simulink library "ddm"  (R2021b)
settings: Solver=VariableStepAuto  StartTime=0.0  StopTime=10.0  RelTol=1e-3
undefined symbols (not defined in the file or in its folder): ENUM_ADASACCSTA_ERROR, ENUM_ADASACCSTA_OFF, ENUM_ADASACCSTA_STANDBY, ENUM_ADASISASTA_OFF, ENUM_ALLOWMOV_ALLOWREADY, ENUM_APS, ENUM_BRKSTA_ERROR, ENUM_BRKSTA_OFF, ENUM_BRKSTA_ON, ENUM_BRKSW_INVALID, ENUM_BRKSW_OFF, ENUM_BRKSW_ON, ENUM_CHGPREACTERRSTA_OBCPRE, ENUM_DCDCFAULTSTA_ANYFAULTLV1, ENUM_DCDCFAULTSTA_ANYFAULTLV2, ENUM_DRIVETRAIN_AWD, ENUM_DRIVETRAIN_FWD, ENUM_DRIVETRAIN_RWD, ENUM_DRSEATSTA_INVALID, ENUM_EDUDRTSTA_NORMAL, ENUM_EPBSTA_APPLIED, ENUM_EPBSTA_RELEASED, ENUM_HVBATTREADYPRE_READY, ENUM_MCUWARN_LV0, ENUM_MCUWARN_LV1, ENUM_MCUWARN_LV2, ENUM_MCUWARN_LV3, ENUM_MCUWARN_NOERROR, ENUM_OBCFAULTSTA_ANYFAULT, ENUM_PAS_R2F2, ENUM_PDFAULT_BATTPDFAIL, ENUM_PDFAULT_DCDCDISABLE, ENUM_PDFAULT_MCUDISABLE, ENUM_PDFAULT_MCUDISCHRG, ENUM_POWERSTA_OFF, ENUM_POWERSTA_ON, ENUM_POWERSTA_READY, ENUM_POWERSTA_STANDBY, ENUM_PRESSINDI_LOW, ENUM_PUFAULT_BATTUPFAIL, ENUM_PUFAULT_DCDCENABLEFAIL, ENUM_PUFAULT_PRECHRGCHKFAIL, ENUM_PUFAULT_SAFETYCHKFAIL, ENUM_PUSTATE_COMPLETED, ENUM_PWRSTASW_OFF, ENUM_PWRSTASW_OFFA, ENUM_PWRSTASW_OFFCHVCHRG, ENUM_PWRSTASW_OFFCLVCHRG, ENUM_PWRSTASW_ON, ENUM_PWRSTASW_ONHVCHRG, ENUM_PWRSTASW_READY, ENUM_PWRSTASW_STANDBY, ENUM_RANGESTA_12IN, ENUM_SHIFTCOMMAND_D, ENUM_SHIFTCOMMAND_N, ENUM_SHIFTCOMMAND_P, ENUM_SHIFTCOMMAND_R, ENUM_VEHMALFUNLV_2ND, ENUM_VEHMALFUNLV_3RD, ENUM_VEHMALFUNLV_4TH ... (+835)
libraries: hcu_lib x750, $bdroot x12, simulink x5
(part 11 of 28)

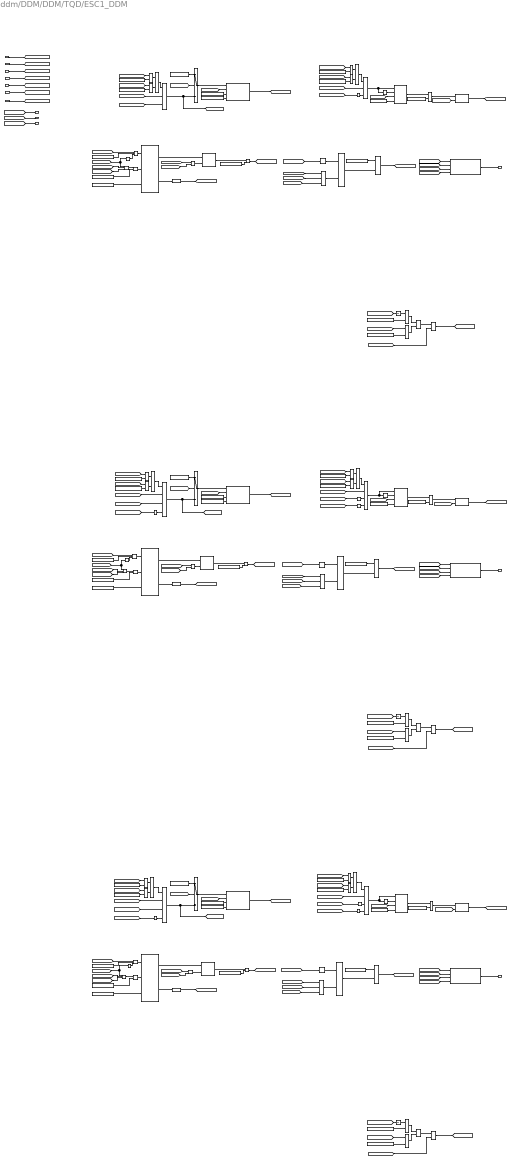
== system ddm/DDM/DDM/TQD/ESC1_DDM ==
  note: ESC1 Lost Comm (ESC1NoCom)
  note: ESC1 Rolling Count Error (ESC1RCErr)
  note: ESC1 CheckSum Error (ESC1CSErr)
  task_time_s : Inport
  VPMM_SysPwrSta_enum : Inport  Port=2
  No_CAN1_BUS_OFF : Inport  Port=3
  VDDM_ESC1NoCom_flg : Inport  Port=4
  VDDM_ESC1RCErr_flg : Inport  Port=5
  VDDM_ESC1CSErr_flg : Inport  Port=6
  DTC_clear_request : Inport  Port=7
  Constant{1,4,6,11,16..17} (6 alike) : Constant  Value=ENUM_PWRSTASW_READY
  Constant10 : Constant  Value=KDDM_ESC1RCErrDFSSW_flg
  Constant12 : Constant  Value=FALSE
  Constant13 : Constant  Value=KDDM_ESC1RCErrDTC_cnt
  Constant14 : Constant  Value=KDDM_ESC1RCErrPassTO_s
  Constant{2..3,5,7,15,19} (6 alike) : Constant  Value=ENUM_PWRSTASW_ON
  Constant18 : Constant  Value=KDDM_ESC1NoComDFSSW_flg
  Constant25 : Constant  Value=KDDM_ESC1RCErrDetTO_s
  Constant27 : Constant  Value=FALSE
  Constant28 : Constant  Value=KDDM_ESC1NoComDTC_cnt
  Constant29 : Constant  Value=KDDM_ESC1NoComPassTO_s
  Constant30 : Constant  Value=KDDM_ESC1NoComDetTO_s
  Constant31 : Constant  Value=ENUM_POWERSTA_OFF
  Constant32 : Constant  Value=ENUM_POWERSTA_STANDBY
  Constant33 : Constant  Value=KDDM_ESC1RCErrDetSW_flg
  Constant34 : Constant  Value=KDDM_ESC1RCErrPassSW_flg
  Constant35 : Constant  Value=KDDM_ESC1RCErrPassTO_s
  Constant36 : Constant  Value=KDDM_ESC1CSErrCFSSW_flg
  Constant37 : Constant  Value=KDDM_ESC1CSErrDTC_cnt
  Constant39 : Constant  Value=KDDM_ESC1CSErrDFSSW_flg
  Constant41 : Constant  Value=FALSE
  Constant42 : Constant  Value=KDDM_ESC1CSErrDTC_cnt
  Constant43 : Constant  Value=KDDM_ESC1CSErrPassTO_s
  Constant44 : Constant  Value=KDDM_ESC1CSErrDetTO_s
  Constant46 : Constant  Value=ENUM_POWERSTA_OFF
  Constant47 : Constant  Value=ENUM_POWERSTA_STANDBY
  Constant48 : Constant  Value=KDDM_ESC1CSErrDetSW_flg
  Constant49 : Constant  Value=ENUM_POWERSTA_OFF
  Constant50 : Constant  Value=KDDM_ESC1CSErrPassSW_flg
  Constant51 : Constant  Value=KDDM_ESC1CSErrPassTO_s
  Constant52 : Constant  Value=ENUM_POWERSTA_STANDBY
  Constant53 : Constant  Value=KDDM_ESC1NoComDetSW_flg
  Constant54 : Constant  Value=KDDM_ESC1NoComPassSW_flg
  Constant55 : Constant  Value=KDDM_ESC1NoComPassTO_s
  Constant56 : Constant  Value=KDDM_ESC1RCErrCFSSW_flg
  Constant57 : Constant  Value=KDDM_ESC1RCErrDTC_cnt
  Constant8 : Constant  Value=KDDM_ESC1NoComCFSSW_flg
  Constant9 : Constant  Value=KDDM_ESC1NoComDTC_cnt
  DTC_Couter2 : hcu_lib/Basic_Blocks/DTC_Couter
  DTC_Couter3 : hcu_lib/Basic_Blocks/DTC_Couter
  DTC_Couter4 : hcu_lib/Basic_Blocks/DTC_Couter
  DTC_Info1 : hcu_lib/Basic_Blocks/DTC_Info
  DTC_Info2 : hcu_lib/Basic_Blocks/DTC_Info
  DTC_Info3 : hcu_lib/Basic_Blocks/DTC_Info
  Data Type Conversion1 : DataTypeConversion  OutDataTypeStr=uint8
  Data Type Conversion3 : DataTypeConversion  OutDataTypeStr=uint8
  Data Type Conversion4 : DataTypeConversion  OutDataTypeStr=uint8
  Equal{1..14,16..18,22} (18 alike) : RelationalOperator  Operator===  OutDataTypeStr=boolean  RndMeth=Simplest
  Equal15 : RelationalOperator  OutDataTypeStr=boolean  RndMeth=Simplest
  Equal20 : RelationalOperator  OutDataTypeStr=boolean  RndMeth=Simplest
  Equal21 : RelationalOperator  OutDataTypeStr=boolean  RndMeth=Simplest
  Logical Operator{1..3,6..7,9..10,15,17,31,34,36} (12 alike) : Logic  Operator=OR  AllPortsSameDT=off  OutDataTypeStr=boolean
  Logical Operator{11..14,16,18..19,26,30,37,41,45,53} (13 alike) : Logic  Operator=NOT  AllPortsSameDT=off  OutDataTypeStr=boolean
  Logical Operator{4,20,22,38,50} (5 alike) : Logic  Inputs=3  AllPortsSameDT=off  OutDataTypeStr=boolean
  Logical Operator{8,21,23..25,27,35,39..40,42,48,52} (12 alike) : Logic  AllPortsSameDT=off  OutDataTypeStr=boolean
  Logical Operator{28,32,43,46} (4 alike) : Logic  Inputs=4  AllPortsSameDT=off  OutDataTypeStr=boolean
  Logical Operator{5,29,33,44,47,51} (6 alike) : Logic  Operator=OR  Inputs=3  AllPortsSameDT=off  OutDataTypeStr=boolean
  Relay2 : Relay  OnSwitchValue=ONE_INT  OffSwitchValue=ZERO_INT
  Relay3 : Relay  OnSwitchValue=ONE_INT  OffSwitchValue=ZERO_INT
  Relay4 : Relay  OnSwitchValue=ONE_INT  OffSwitchValue=ZERO_INT
  SR_Latch{3..11} (9 alike) : hcu_lib/Basic_Blocks/SR_Latch
  Switch1 : Switch  Criteria=u2 ~= 0
  Switch2 : Switch  Criteria=u2 ~= 0
  Switch3 : Switch  Criteria=u2 ~= 0
  Test Detection Criteria2 : hcu_lib/Basic_Blocks/Test Detection Criteria
  Test Detection Criteria3 : hcu_lib/Basic_Blocks/Test Detection Criteria
  Test Detection Criteria4 : hcu_lib/Basic_Blocks/Test Detection Criteria
  Timer1 : hcu_lib/Basic_Blocks/Timer
  Timer3 : hcu_lib/Basic_Blocks/Timer
  Timer4 : hcu_lib/Basic_Blocks/Timer
  Unit Delay1 : UnitDelay  SampleTime=-1  HasFrameUpgradeWarning=on
  Unit Delay3 : UnitDelay  SampleTime=-1  HasFrameUpgradeWarning=on
  Unit Delay4 : UnitDelay  SampleTime=-1  HasFrameUpgradeWarning=on
  VDDM_ESC1NoComDTC_raw32 : Outport
  VDDM_ESC1RCErrDTC_raw32 : Outport  Port=2
  VDDM_ESC1CSErrDTC_raw32 : Outport  Port=3
  VDDM_ESC1NoComCFS_flg : Outport  Port=4
  VDDM_ESC1RCErrCFS_flg : Outport  Port=5
  VDDM_ESC1CSErrCFS_flg : Outport  Port=6
  wires:
  Constant5/1 -> Equal11/2
  [VDDM_ESC1CSErr_flg] -> Logical Operator32/3
  Logical Operator5/1 -> Logical Operator21/1
  [VDDM_ESC1RCErrPass_flg] -> Logical Operator47/2
  Logical Operator23/1 -> DTC_Couter3/2
  [VDDM_ESC1CSErrCFSRls_flg] -> Logical Operator33/3
  Constant53/1 -> Logical Operator20/2
  Equal21/1 -> SR_Latch7/1
  Constant55/1 -> Timer3/4
  Timer3/1 -> Equal20/1
  Logical Operator36/1 -> [VDDM_ESC1RCErrCFSRls_flg]  "VDDM_ESC1RCErrCFSRls_flg"
  Constant33/1 -> Logical Operator22/2
  [DTC_clear_request] -> DTC_Info1/4
  Equal10/1 -> Logical Operator2/2
  Constant50/1 -> Logical Operator39/2
  Constant18/1 -> Logical Operator48/1
  [VPMM_SysPwrSta_enum] -> Unit Delay3/1
  [No_CAN1_BUS_OFF] -> Logical Operator46/2
  Constant41/1 -> Switch2/1
  Logical Operator45/1 -> Logical Operator43/3
  Constant29/1 -> Equal20/2
  Equal1/1 -> Logical Operator52/1
  Logical Operator40/1 -> [VDDM_ESC1CSErrCFS_flg]  "VDDM_ESC1CSErrCFS_flg"
  Constant47/1 -> Equal5/2
  Constant27/1 -> Switch3/1
  Equal16/1 -> Logical Operator52/2
  task_time_s/1 -> [task_time_s]
  Logical Operator10/1 -> Logical Operator43/1
  DTC_Info2/1 -> VDDM_ESC1RCErrDTC_raw32/1  "VDDM_ESC1RCErrDTC_raw32"
  Constant32/1 -> Equal16/2
  [DTC_clear_request] -> Logical Operator31/2
  Logical Operator25/1 -> [VDDM_ESC1NoComCFS_flg]  "VDDM_ESC1NoComCFS_flg"
  Constant46/1 -> Equal22/2
  [VDDM_ESC1CSErr_flg] -> Logical Operator45/1
  Equal20/1 -> SR_Latch4/1
  Relay3/1 -> SR_Latch8/1
  [No_CAN1_BUS_OFF] -> Logical Operator43/2
  [VDDM_ESC1NoComCFS_flg] -> DTC_Info1/3
  SR_Latch6/1 -> Logical Operator24/1
  [task_time_s] -> Test Detection Criteria2/2
  DTC_Info3/1 -> VDDM_ESC1CSErrDTC_raw32/1  "VDDM_ESC1CSErrDTC_raw32"
  [task_time_s] -> Timer3/3
  [VDDM_ESC1NoComPass_flg] -> Logical Operator5/2
  Constant25/1 -> Test Detection Criteria3/4
  [DTC_clear_request] -> DTC_Info2/4
  Equal9/1 -> Logical Operator1/1
  [VPMM_SysPwrSta_enum] -> Unit Delay1/1
  Constant28/1 -> Test Detection Criteria2/3
  [VDDM_ESC1NoComDFSRls_flg] -> Logical Operator51/1
  Data Type Conversion3/1 -> [VDDM_ESC1NoComDTC_cnt]  "VDDM_ESC1NoComDTC_cnt"
  Constant48/1 -> Logical Operator38/2
  [VDDM_ESC1NoComDTC_cnt] -> Relay2/1
  [VPMM_SysPwrSta_enum] -> Equal14/1
  [VDDM_ESC1NoComCFS_flg] -> Logical Operator51/2
  [VDDM_ESC1RCErrRst_flg] -> SR_Latch7/2
  Logical Operator42/1 -> [VDDM_ESC1CSErrDFS_flg]  "VDDM_ESC1CSErrDFS_flg"
  Equal22/1 -> Logical Operator35/1
  [VDDM_ESC1CSErrRst_flg] -> SR_Latch10/2
  Logical Operator47/1 -> Logical Operator23/1
  Constant30/1 -> Test Detection Criteria2/4
  [VPMM_SysPwrSta_enum] -> Equal4/1
  Constant43/1 -> Equal15/2
  Logical Operator20/1 -> DTC_Couter2/1
  SR_Latch10/1 -> [VDDM_ESC1CSErrPass_flg]  "VDDM_ESC1CSErrPass_flg"
  Equal7/1 -> Logical Operator1/2
  [VPMM_SysPwrSta_enum] -> Equal10/1
  [VDDM_ESC1CSErrPass_flg] -> DTC_Info3/2
  Switch2/1 -> Test Detection Criteria4/1
  [VPMM_SysPwrSta_enum] -> Equal7/1
  Constant51/1 -> Timer4/4
  Constant4/1 -> Equal10/2
  Constant19/1 -> Equal18/2
  Logical Operator2/1 -> Logical Operator46/1
  Constant3/1 -> Equal6/2
  [VPMM_SysPwrSta_enum] -> Equal18/1
  Equal6/1 -> Logical Operator9/1
  Constant17/1 -> Equal2/2
  [VPMM_SysPwrSta_enum] -> Equal2/1
  [VPMM_SysPwrSta_enum] -> Equal6/1
  VPMM_SysPwrSta_enum/1 -> [VPMM_SysPwrSta_enum]
  Constant16/1 -> Equal8/2
  [DTC_clear_request] -> Switch3/2
  [VDDM_ESC1CSErrCFSRls_flg] -> Logical Operator17/1
  [VPMM_SysPwrSta_enum] -> Equal8/1
  Unit Delay1/1 -> Equal1/1
  [task_time_s] -> Timer1/3
  Logical Operator44/1 -> SR_Latch11/2
  [DTC_clear_request] -> Logical Operator3/2
  Relay4/1 -> SR_Latch11/1
  [VDDM_ESC1RCErrPass_flg] -> DTC_Info2/2
  [VDDM_ESC1NoComCFSRls_flg] -> Logical Operator5/3
  Constant8/1 -> Logical Operator25/2
  Logical Operator48/1 -> [VDDM_ESC1NoComDFS_flg]  "VDDM_ESC1NoComDFS_flg"
  [VDDM_ESC1RCErrDet_flg] -> Logical Operator22/1
  [VPMM_SysPwrSta_enum] -> Equal13/1
  [VPMM_SysPwrSta_enum] -> Equal12/1
  Logical Operator21/1 -> DTC_Couter2/2
  SR_Latch4/1 -> [VDDM_ESC1NoComPass_flg]  "VDDM_ESC1NoComPass_flg"
  Logical Operator32/1 -> [VDDM_ESC1CSErrRst_flg], Switch2/3
  Constant6/1 -> Equal12/2
  [DTC_clear_request] -> Logical Operator36/2
  Equal13/1 -> Logical Operator6/1
  Constant7/1 -> Equal13/2
  Constant14/1 -> Equal21/2
  [No_CAN1_BUS_OFF] -> Logical Operator28/2
  Equal2/1 -> Logical Operator9/2
  Logical Operator6/1 -> Logical Operator28/1
  Constant31/1 -> Equal1/2
  Constant10/1 -> Logical Operator27/1
  [VPMM_SysPwrSta_enum] -> Equal11/1
  [VDDM_ESC1NoComDet_flg] -> DTC_Info1/1
  Timer1/1 -> Equal21/1
  Data Type Conversion1/1 -> [VDDM_ESC1RCErrDTC_cnt]  "VDDM_ESC1RCErrDTC_cnt"
  [VDDM_ESC1NoComDet_flg] -> Logical Operator20/1
  Logical Operator27/1 -> [VDDM_ESC1RCErrDFS_flg]  "VDDM_ESC1RCErrDFS_flg"
  Logical Operator8/1 -> Logical Operator3/1
  Logical Operator30/1 -> Logical Operator28/3
  Constant35/1 -> Timer1/4
  [VDDM_ESC1RCErrCFS_flg] -> DTC_Info2/3
  Logical Operator33/1 -> Logical Operator39/1
  DTC_clear_request/1 -> [DTC_clear_request]
  Equal3/1 -> Logical Operator8/1
  [VPMM_SysPwrSta_enum] -> Equal17/1
  Logical Operator35/1 -> Logical Operator31/1
  [VDDM_ESC1NoComRst_flg] -> SR_Latch4/2
  [VDDM_ESC1NoComCFS_flg] -> Logical Operator41/1
  Constant42/1 -> Test Detection Criteria4/3
  [DTC_clear_request] -> Switch2/2
  Logical Operator1/1 -> Logical Operator50/1
  SR_Latch3/1 -> Logical Operator25/1
  SR_Latch8/1 -> Logical Operator27/2
  [DTC_clear_request] -> DTC_Info3/4
  [VPMM_SysPwrSta_enum] -> Equal5/1
  Constant56/1 -> Logical Operator24/2
  Equal8/1 -> Logical Operator10/2
  [VDDM_ESC1NoComCFS_flg] -> Logical Operator26/1
  Logical Operator29/1 -> SR_Latch8/2
  [VPMM_SysPwrSta_enum] -> Unit Delay4/1
  [VDDM_ESC1CSErrDTC_cnt] -> Relay4/1
  No_CAN1_BUS_OFF/1 -> [No_CAN1_BUS_OFF]
  Logical Operator50/1 -> Logical Operator19/1, Timer3/1
  [VDDM_ESC1CSErrDet_flg] -> DTC_Info3/1
  Data Type Conversion4/1 -> [VDDM_ESC1CSErrDTC_cnt]  "VDDM_ESC1CSErrDTC_cnt"
  Equal15/1 -> SR_Latch10/1
  Logical Operator7/1 -> Logical Operator32/1
  [VDDM_ESC1RCErr_flg] -> Logical Operator46/3
  Switch1/1 -> Test Detection Criteria3/1
  [VDDM_ESC1RCErrCFSRls_flg] -> Logical Operator47/3
  Test Detection Criteria4/1 -> [VDDM_ESC1CSErrDet_flg]  "VDDM_ESC1CSErrDet_flg"
  Constant13/1 -> Test Detection Criteria3/3
  DTC_Info1/1 -> VDDM_ESC1NoComDTC_raw32/1  "VDDM_ESC1NoComDTC_raw32"
  Constant36/1 -> Logical Operator40/2
  [VDDM_ESC1CSErrCFS_flg] -> Logical Operator44/2
  Logical Operator9/1 -> Logical Operator4/1
  DTC_Couter2/2 -> Data Type Conversion3/1
  Logical Operator51/1 -> SR_Latch5/2
  Logical Operator28/1 -> Timer1/1, Logical Operator12/1
  Logical Operator39/1 -> DTC_Couter4/2
  Logical Operator31/1 -> [VDDM_ESC1CSErrCFSRls_flg]  "VDDM_ESC1CSErrCFSRls_flg"
  Logical Operator3/1 -> [VDDM_ESC1NoComCFSRls_flg]  "VDDM_ESC1NoComCFSRls_flg"
  [VDDM_ESC1RCErrCFS_flg] -> Logical Operator29/2
  [VDDM_ESC1RCErrDTC_cnt] -> Relay3/1
  Relay2/1 -> SR_Latch5/1
  [task_time_s] -> Test Detection Criteria4/2
  Logical Operator38/1 -> DTC_Couter4/1
  [VDDM_ESC1RCErrDet_flg] -> DTC_Info2/1
  [task_time_s] -> Test Detection Criteria3/2
  Logical Operator24/1 -> [VDDM_ESC1RCErrCFS_flg]  "VDDM_ESC1RCErrCFS_flg"
  Logical Operator4/1 -> [VDDM_ESC1NoComRst_flg], Switch3/3
  [VPMM_SysPwrSta_enum] -> Equal9/1
  Constant11/1 -> Equal14/2
  [No_CAN1_BUS_OFF] -> Logical Operator4/2
  Equal18/1 -> Logical Operator10/1
  Logical Operator12/1 -> Timer1/2
  Constant12/1 -> Switch1/1
  [task_time_s] -> Timer4/3
  Equal5/1 -> Logical Operator35/2
  Equal17/1 -> Logical Operator7/1
  Equal11/1 -> Logical Operator2/1
  DTC_Couter3/1 -> SR_Latch6/1
  Equal12/1 -> Logical Operator6/2
  Unit Delay3/1 -> Equal3/1
  SR_Latch9/1 -> Logical Operator40/1
  Equal14/1 -> Logical Operator7/2
  [DTC_clear_request] -> Switch1/2
  Constant52/1 -> Equal4/2
  [VDDM_ESC1NoComCFSRls_flg] -> Logical Operator34/1
  Logical Operator26/1 -> Logical Operator46/4
  Constant57/1 -> DTC_Couter3/3
  [VDDM_ESC1CSErrCFS_flg] -> DTC_Info3/3
  Constant1/1 -> Equal7/2
  Constant39/1 -> Logical Operator42/1
  [VDDM_ESC1CSErrDFSRls_flg] -> Logical Operator44/1
  Constant44/1 -> Test Detection Criteria4/4
  Logical Operator46/1 -> [VDDM_ESC1RCErrRst_flg], Switch1/3
  Logical Operator22/1 -> DTC_Couter3/1
  Logical Operator53/1 -> Logical Operator50/3
  Constant37/1 -> DTC_Couter4/3
  DTC_Couter4/2 -> Data Type Conversion4/1
  DTC_Couter3/2 -> Data Type Conversion1/1
  Constant9/1 -> DTC_Couter2/3
  DTC_Couter2/1 -> SR_Latch3/1
  Constant2/1 -> Equal9/2
  Logical Operator43/1 -> Timer4/1, Logical Operator37/1
  Unit Delay4/1 -> Equal22/1
  SR_Latch7/1 -> [VDDM_ESC1RCErrPass_flg]  "VDDM_ESC1RCErrPass_flg"
  Logical Operator19/1 -> Timer3/2
  Constant15/1 -> Equal17/2
  [VDDM_ESC1RCErr_flg] -> Logical Operator30/1
  Logical Operator41/1 -> Logical Operator32/4
  Timer4/1 -> Equal15/1
  Switch3/1 -> Test Detection Criteria2/1
  Logical Operator52/1 -> Logical Operator36/1
  [VDDM_ESC1CSErrDet_flg] -> Logical Operator38/1
  VDDM_ESC1NoCom_flg/1 -> [VDDM_ESC1NoCom_flg]
  [VDDM_ESC1NoComPass_flg] -> DTC_Info1/2
  [VDDM_ESC1NoCom_flg] -> Logical Operator53/1
  [No_CAN1_BUS_OFF] -> Logical Operator50/2
  [No_CAN1_BUS_OFF] -> Logical Operator32/2
  [VPMM_SysPwrSta_enum] -> Equal16/1
  SR_Latch11/1 -> Logical Operator42/2
  Test Detection Criteria3/1 -> [VDDM_ESC1RCErrDet_flg]  "VDDM_ESC1RCErrDet_flg"
  [VDDM_ESC1CSErrPass_flg] -> Logical Operator33/2
  [VDDM_ESC1RCErrCFSRls_flg] -> Logical Operator15/1
  Equal4/1 -> Logical Operator8/2
  DTC_Couter4/1 -> SR_Latch9/1
  Logical Operator37/1 -> Timer4/2
  SR_Latch5/1 -> Logical Operator48/2
  Constant54/1 -> Logical Operator21/2
  Test Detection Criteria2/1 -> [VDDM_ESC1NoComDet_flg]  "VDDM_ESC1NoComDet_flg"
  Constant34/1 -> Logical Operator23/2
  [VDDM_ESC1NoCom_flg] -> Logical Operator4/3
  Constant49/1 -> Equal3/2
  [VDDM_ESC1RCErrDFSRls_flg] -> Logical Operator29/1
  VDDM_ESC1RCErr_flg/1 -> [VDDM_ESC1RCErr_flg]
  VDDM_ESC1CSErr_flg/1 -> [VDDM_ESC1CSErr_flg]
  Logical Operator11/1 -> Logical Operator28/4
  [VDDM_ESC1NoComCFS_flg] -> Logical Operator11/1
  Logical Operator13/1 -> Logical Operator43/4
  [VDDM_ESC1NoComCFS_flg] -> Logical Operator13/1
  [VDDM_ESC1NoComCFS_flg] -> VDDM_ESC1NoComCFS_flg/1
  [VDDM_ESC1CSErrCFS_flg] -> VDDM_ESC1CSErrCFS_flg/1
  [VDDM_ESC1RCErrCFS_flg] -> VDDM_ESC1RCErrCFS_flg/1
  Logical Operator14/1 -> Logical Operator22/3
  [DTC_clear_request] -> Logical Operator47/1, Logical Operator14/1
  [DTC_clear_request] -> Logical Operator15/2
  Logical Operator15/1 -> SR_Latch6/2
  [DTC_clear_request] -> Logical Operator29/3
  Logical Operator16/1 -> Logical Operator38/3
  [DTC_clear_request] -> Logical Operator33/1, Logical Operator16/1
  Logical Operator17/1 -> SR_Latch9/2
  [DTC_clear_request] -> Logical Operator17/2
  [DTC_clear_request] -> Logical Operator44/3
  Logical Operator18/1 -> Logical Operator20/3
  [DTC_clear_request] -> Logical Operator5/1, Logical Operator18/1
  Logical Operator34/1 -> SR_Latch3/2
  [DTC_clear_request] -> Logical Operator34/2
  [DTC_clear_request] -> Logical Operator51/3

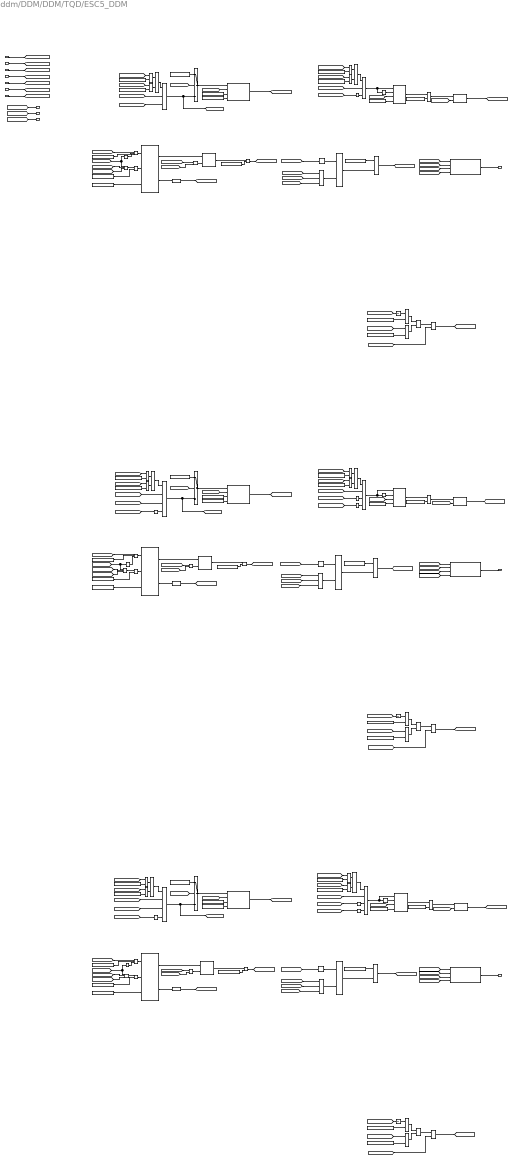
== system ddm/DDM/DDM/TQD/ESC5_DDM ==
  note: ESC5 Lost Comm (ESC5NoCom)
  note: ESC5 Rolling Count Error (ESC5RCErr)
  note: ESC5 CheckSum Error (ESC5CSErr)
  task_time_s : Inport
  VPMM_SysPwrSta_enum : Inport  Port=2
  No_CAN1_BUS_OFF : Inport  Port=3
  VDDM_ESC5NoCom_flg : Inport  Port=4
  VDDM_ESC5RCErr_flg : Inport  Port=5
  VDDM_ESC5CSErr_flg : Inport  Port=6
  DTC_clear_request : Inport  Port=7
  Constant{1,4,6,11,16..17} (6 alike) : Constant  Value=ENUM_PWRSTASW_READY
  Constant10 : Constant  Value=KDDM_ESC5RCErrDFSSW_flg
  Constant12 : Constant  Value=FALSE
  Constant13 : Constant  Value=KDDM_ESC5RCErrDTC_cnt
  Constant14 : Constant  Value=KDDM_ESC5RCErrPassTO_s
  Constant{2..3,5,7,15,19} (6 alike) : Constant  Value=ENUM_PWRSTASW_ON
  Constant18 : Constant  Value=KDDM_ESC5NoComDFSSW_flg
  Constant25 : Constant  Value=KDDM_ESC5RCErrDetTO_s
  Constant27 : Constant  Value=FALSE
  Constant28 : Constant  Value=KDDM_ESC5NoComDTC_cnt
  Constant29 : Constant  Value=KDDM_ESC5NoComPassTO_s
  Constant30 : Constant  Value=KDDM_ESC5NoComDetTO_s
  Constant31 : Constant  Value=ENUM_POWERSTA_OFF
  Constant32 : Constant  Value=ENUM_POWERSTA_STANDBY
  Constant33 : Constant  Value=KDDM_ESC5RCErrDetSW_flg
  Constant34 : Constant  Value=KDDM_ESC5RCErrPassSW_flg
  Constant35 : Constant  Value=KDDM_ESC5RCErrPassTO_s
  Constant36 : Constant  Value=KDDM_ESC5CSErrCFSSW_flg
  Constant37 : Constant  Value=KDDM_ESC5CSErrDTC_cnt
  Constant39 : Constant  Value=KDDM_ESC5CSErrDFSSW_flg
  Constant41 : Constant  Value=FALSE
  Constant42 : Constant  Value=KDDM_ESC5CSErrDTC_cnt
  Constant43 : Constant  Value=KDDM_ESC5CSErrPassTO_s
  Constant44 : Constant  Value=KDDM_ESC5CSErrDetTO_s
  Constant46 : Constant  Value=ENUM_POWERSTA_OFF
  Constant47 : Constant  Value=ENUM_POWERSTA_STANDBY
  Constant48 : Constant  Value=KDDM_ESC5CSErrDetSW_flg
  Constant49 : Constant  Value=ENUM_POWERSTA_OFF
  Constant50 : Constant  Value=KDDM_ESC5CSErrPassSW_flg
  Constant51 : Constant  Value=KDDM_ESC5CSErrPassTO_s
  Constant52 : Constant  Value=ENUM_POWERSTA_STANDBY
  Constant53 : Constant  Value=KDDM_ESC5NoComDetSW_flg
  Constant54 : Constant  Value=KDDM_ESC5NoComPassSW_flg
  Constant55 : Constant  Value=KDDM_ESC5NoComPassTO_s
  Constant56 : Constant  Value=KDDM_ESC5RCErrCFSSW_flg
  Constant57 : Constant  Value=KDDM_ESC5RCErrDTC_cnt
  Constant8 : Constant  Value=KDDM_ESC5NoComCFSSW_flg
  Constant9 : Constant  Value=KDDM_ESC5NoComDTC_cnt
  DTC_Couter2 : hcu_lib/Basic_Blocks/DTC_Couter
  DTC_Couter3 : hcu_lib/Basic_Blocks/DTC_Couter
  DTC_Couter4 : hcu_lib/Basic_Blocks/DTC_Couter
  DTC_Info1 : hcu_lib/Basic_Blocks/DTC_Info
  DTC_Info2 : hcu_lib/Basic_Blocks/DTC_Info
  DTC_Info3 : hcu_lib/Basic_Blocks/DTC_Info
  Data Type Conversion1 : DataTypeConversion  OutDataTypeStr=uint8
  Data Type Conversion3 : DataTypeConversion  OutDataTypeStr=uint8
  Data Type Conversion4 : DataTypeConversion  OutDataTypeStr=uint8
  Equal{1..14,16..18,22} (18 alike) : RelationalOperator  Operator===  OutDataTypeStr=boolean  RndMeth=Simplest
  Equal15 : RelationalOperator  OutDataTypeStr=boolean  RndMeth=Simplest
  Equal20 : RelationalOperator  OutDataTypeStr=boolean  RndMeth=Simplest
  Equal21 : RelationalOperator  OutDataTypeStr=boolean  RndMeth=Simplest
  Logical Operator{1..3,6..7,9..10,14,17,31,34,36} (12 alike) : Logic  Operator=OR  AllPortsSameDT=off  OutDataTypeStr=boolean
  Logical Operator{11..13,15..16,18..19,26,30,37,41,45,53} (13 alike) : Logic  Operator=NOT  AllPortsSameDT=off  OutDataTypeStr=boolean
  Logical Operator{4,20,22,38,50} (5 alike) : Logic  Inputs=3  AllPortsSameDT=off  OutDataTypeStr=boolean
  Logical Operator{8,21,23..25,27,35,39..40,42,48,52} (12 alike) : Logic  AllPortsSameDT=off  OutDataTypeStr=boolean
  Logical Operator{28,32,43,46} (4 alike) : Logic  Inputs=4  AllPortsSameDT=off  OutDataTypeStr=boolean
  Logical Operator{5,29,33,44,47,51} (6 alike) : Logic  Operator=OR  Inputs=3  AllPortsSameDT=off  OutDataTypeStr=boolean
  Relay2 : Relay  OnSwitchValue=ONE_INT  OffSwitchValue=ZERO_INT
  Relay3 : Relay  OnSwitchValue=ONE_INT  OffSwitchValue=ZERO_INT
  Relay4 : Relay  OnSwitchValue=ONE_INT  OffSwitchValue=ZERO_INT
  SR_Latch{3..11} (9 alike) : hcu_lib/Basic_Blocks/SR_Latch
  Switch1 : Switch  Criteria=u2 ~= 0
  Switch2 : Switch  Criteria=u2 ~= 0
  Switch3 : Switch  Criteria=u2 ~= 0
  Test Detection Criteria2 : hcu_lib/Basic_Blocks/Test Detection Criteria
  Test Detection Criteria3 : hcu_lib/Basic_Blocks/Test Detection Criteria
  Test Detection Criteria4 : hcu_lib/Basic_Blocks/Test Detection Criteria
  Timer1 : hcu_lib/Basic_Blocks/Timer
  Timer3 : hcu_lib/Basic_Blocks/Timer
  Timer4 : hcu_lib/Basic_Blocks/Timer
  Unit Delay1 : UnitDelay  SampleTime=-1  HasFrameUpgradeWarning=on
  Unit Delay3 : UnitDelay  SampleTime=-1  HasFrameUpgradeWarning=on
  Unit Delay4 : UnitDelay  SampleTime=-1  HasFrameUpgradeWarning=on
  VDDM_ESC5NoComDTC_raw32 : Outport
  VDDM_ESC5RCErrDTC_raw32 : Outport  Port=2
  VDDM_ESC5CSErrDTC_raw32 : Outport  Port=3
  VDDM_ESC5NoComCFS_flg : Outport  Port=4
  VDDM_ESC5RCErrCFS_flg : Outport  Port=5
  VDDM_ESC5CSErrCFS_flg : Outport  Port=6
  wires:
  Constant5/1 -> Equal11/2
  [VDDM_ESC5CSErr_flg] -> Logical Operator32/3
  Logical Operator5/1 -> Logical Operator21/1
  [VDDM_ESC5RCErrPass_flg] -> Logical Operator47/2
  Logical Operator23/1 -> DTC_Couter3/2
  [VDDM_ESC5CSErrCFSRls_flg] -> Logical Operator33/3
  Constant53/1 -> Logical Operator20/2
  Equal21/1 -> SR_Latch7/1
  Constant55/1 -> Timer3/4
  Timer3/1 -> Equal20/1
  Logical Operator36/1 -> [VDDM_ESC5RCErrCFSRls_flg]  "VDDM_ESC5RCErrCFSRls_flg"
  Constant33/1 -> Logical Operator22/2
  [DTC_clear_request] -> DTC_Info1/4
  Equal10/1 -> Logical Operator2/2
  Constant50/1 -> Logical Operator39/2
  Constant18/1 -> Logical Operator48/1
  [VPMM_SysPwrSta_enum] -> Unit Delay3/1
  [No_CAN1_BUS_OFF] -> Logical Operator46/2
  Constant41/1 -> Switch2/1
  Logical Operator45/1 -> Logical Operator43/3
  Constant29/1 -> Equal20/2
  Equal1/1 -> Logical Operator52/1
  Logical Operator40/1 -> [VDDM_ESC5CSErrCFS_flg]  "VDDM_ESC5CSErrCFS_flg"
  Constant47/1 -> Equal5/2
  Constant27/1 -> Switch3/1
  Equal16/1 -> Logical Operator52/2
  task_time_s/1 -> [task_time_s]
  Logical Operator10/1 -> Logical Operator43/1
  DTC_Info2/1 -> VDDM_ESC5RCErrDTC_raw32/1  "VDDM_ESC5RCErrDTC_raw32"
  Constant32/1 -> Equal16/2
  [DTC_clear_request] -> Logical Operator31/2
  Logical Operator25/1 -> [VDDM_ESC5NoComCFS_flg]  "VDDM_ESC5NoComCFS_flg"
  Constant46/1 -> Equal22/2
  [VDDM_ESC5CSErr_flg] -> Logical Operator45/1
  Equal20/1 -> SR_Latch4/1
  Relay3/1 -> SR_Latch8/1
  [No_CAN1_BUS_OFF] -> Logical Operator43/2
  [VDDM_ESC5NoComCFS_flg] -> DTC_Info1/3
  SR_Latch6/1 -> Logical Operator24/1
  [task_time_s] -> Test Detection Criteria2/2
  DTC_Info3/1 -> VDDM_ESC5CSErrDTC_raw32/1  "VDDM_ESC5CSErrDTC_raw32"
  [task_time_s] -> Timer3/3
  [VDDM_ESC5NoComPass_flg] -> Logical Operator5/2
  Constant25/1 -> Test Detection Criteria3/4
  [DTC_clear_request] -> DTC_Info2/4
  Equal9/1 -> Logical Operator1/1
  [VPMM_SysPwrSta_enum] -> Unit Delay1/1
  Constant28/1 -> Test Detection Criteria2/3
  [VDDM_ESC5NoComDFSRls_flg] -> Logical Operator51/1
  Data Type Conversion3/1 -> [VDDM_ESC5NoComDTC_cnt]  "VDDM_ESC5NoComDTC_cnt"
  Constant48/1 -> Logical Operator38/2
  [VDDM_ESC5NoComDTC_cnt] -> Relay2/1
  [VPMM_SysPwrSta_enum] -> Equal14/1
  [VDDM_ESC5NoComCFS_flg] -> Logical Operator51/2
  [VDDM_ESC5RCErrRst_flg] -> SR_Latch7/2
  Logical Operator42/1 -> [VDDM_ESC5CSErrDFS_flg]  "VDDM_ESC5CSErrDFS_flg"
  Equal22/1 -> Logical Operator35/1
  Logical Operator47/1 -> Logical Operator23/1
  Constant30/1 -> Test Detection Criteria2/4
  [VPMM_SysPwrSta_enum] -> Equal4/1
  Constant43/1 -> Equal15/2
  Logical Operator20/1 -> DTC_Couter2/1
  SR_Latch10/1 -> [VDDM_ESC5CSErrPass_flg]  "VDDM_ESC5CSErrPass_flg"
  Equal7/1 -> Logical Operator1/2
  [VPMM_SysPwrSta_enum] -> Equal10/1
  [VDDM_ESC5CSErrPass_flg] -> DTC_Info3/2
  Switch2/1 -> Test Detection Criteria4/1
  [VPMM_SysPwrSta_enum] -> Equal7/1
  Constant51/1 -> Timer4/4
  Constant4/1 -> Equal10/2
  Constant19/1 -> Equal18/2
  Logical Operator2/1 -> Logical Operator46/1
  Constant3/1 -> Equal6/2
  [VPMM_SysPwrSta_enum] -> Equal18/1
  Equal6/1 -> Logical Operator9/1
  Constant17/1 -> Equal2/2
  [VPMM_SysPwrSta_enum] -> Equal2/1
  [VPMM_SysPwrSta_enum] -> Equal6/1
  VPMM_SysPwrSta_enum/1 -> [VPMM_SysPwrSta_enum]
  Constant16/1 -> Equal8/2
  [DTC_clear_request] -> Switch3/2
  [VDDM_ESC5CSErrCFSRls_flg] -> Logical Operator34/1
  [VPMM_SysPwrSta_enum] -> Equal8/1
  Unit Delay1/1 -> Equal1/1
  [task_time_s] -> Timer1/3
  Logical Operator44/1 -> SR_Latch11/2
  [DTC_clear_request] -> Logical Operator3/2
  Relay4/1 -> SR_Latch11/1
  [VDDM_ESC5RCErrPass_flg] -> DTC_Info2/2
  [VDDM_ESC5NoComCFSRls_flg] -> Logical Operator5/3
  Constant8/1 -> Logical Operator25/2
  Logical Operator48/1 -> [VDDM_ESC5NoComDFS_flg]  "VDDM_ESC5NoComDFS_flg"
  [VDDM_ESC5RCErrDet_flg] -> Logical Operator22/1
  [VPMM_SysPwrSta_enum] -> Equal13/1
  [VPMM_SysPwrSta_enum] -> Equal12/1
  Logical Operator21/1 -> DTC_Couter2/2
  SR_Latch4/1 -> [VDDM_ESC5NoComPass_flg]  "VDDM_ESC5NoComPass_flg"
  Logical Operator32/1 -> [VDDM_ESC5CSErrRst_flg], Switch2/3
  Constant6/1 -> Equal12/2
  [DTC_clear_request] -> Logical Operator36/2
  Equal13/1 -> Logical Operator6/1
  Constant7/1 -> Equal13/2
  Constant14/1 -> Equal21/2
  [No_CAN1_BUS_OFF] -> Logical Operator28/2
  Equal2/1 -> Logical Operator9/2
  Logical Operator6/1 -> Logical Operator28/1
  Constant31/1 -> Equal1/2
  Constant10/1 -> Logical Operator27/1
  [VPMM_SysPwrSta_enum] -> Equal11/1
  [VDDM_ESC5NoComDet_flg] -> DTC_Info1/1
  Timer1/1 -> Equal21/1
  Data Type Conversion1/1 -> [VDDM_ESC5RCErrDTC_cnt]  "VDDM_ESC5RCErrDTC_cnt"
  [VDDM_ESC5NoComDet_flg] -> Logical Operator20/1
  Logical Operator27/1 -> [VDDM_ESC5RCErrDFS_flg]  "VDDM_ESC5RCErrDFS_flg"
  Logical Operator8/1 -> Logical Operator3/1
  Logical Operator30/1 -> Logical Operator28/3
  Constant35/1 -> Timer1/4
  [VDDM_ESC5RCErrCFS_flg] -> DTC_Info2/3
  Logical Operator33/1 -> Logical Operator39/1
  DTC_clear_request/1 -> [DTC_clear_request]
  Equal3/1 -> Logical Operator8/1
  [VPMM_SysPwrSta_enum] -> Equal17/1
  Logical Operator35/1 -> Logical Operator31/1
  [VDDM_ESC5NoComRst_flg] -> SR_Latch4/2
  [VDDM_ESC5NoComCFS_flg] -> Logical Operator41/1
  Constant42/1 -> Test Detection Criteria4/3
  [DTC_clear_request] -> Switch2/2
  Logical Operator1/1 -> Logical Operator50/1
  SR_Latch3/1 -> Logical Operator25/1
  SR_Latch8/1 -> Logical Operator27/2
  [DTC_clear_request] -> DTC_Info3/4
  [VPMM_SysPwrSta_enum] -> Equal5/1
  Constant56/1 -> Logical Operator24/2
  Equal8/1 -> Logical Operator10/2
  [VDDM_ESC5NoComCFS_flg] -> Logical Operator26/1
  Logical Operator29/1 -> SR_Latch8/2
  [VPMM_SysPwrSta_enum] -> Unit Delay4/1
  [VDDM_ESC5CSErrDTC_cnt] -> Relay4/1
  No_CAN1_BUS_OFF/1 -> [No_CAN1_BUS_OFF]
  Logical Operator50/1 -> Logical Operator19/1, Timer3/1
  [VDDM_ESC5CSErrDet_flg] -> DTC_Info3/1
  Data Type Conversion4/1 -> [VDDM_ESC5CSErrDTC_cnt]  "VDDM_ESC5CSErrDTC_cnt"
  Equal15/1 -> SR_Latch10/1
  Logical Operator7/1 -> Logical Operator32/1
  [VDDM_ESC5RCErr_flg] -> Logical Operator46/3
  Switch1/1 -> Test Detection Criteria3/1
  [VDDM_ESC5RCErrCFSRls_flg] -> Logical Operator47/3
  Test Detection Criteria4/1 -> [VDDM_ESC5CSErrDet_flg]  "VDDM_ESC5CSErrDet_flg"
  Constant13/1 -> Test Detection Criteria3/3
  DTC_Info1/1 -> VDDM_ESC5NoComDTC_raw32/1  "VDDM_ESC5NoComDTC_raw32"
  Constant36/1 -> Logical Operator40/2
  [VDDM_ESC5CSErrCFS_flg] -> Logical Operator44/2
  Logical Operator9/1 -> Logical Operator4/1
  DTC_Couter2/2 -> Data Type Conversion3/1
  Logical Operator51/1 -> SR_Latch5/2
  Logical Operator28/1 -> Timer1/1, Logical Operator12/1
  Logical Operator39/1 -> DTC_Couter4/2
  Logical Operator31/1 -> [VDDM_ESC5CSErrCFSRls_flg]  "VDDM_ESC5CSErrCFSRls_flg"
  Logical Operator3/1 -> [VDDM_ESC5NoComCFSRls_flg]  "VDDM_ESC5NoComCFSRls_flg"
  [VDDM_ESC5RCErrCFS_flg] -> Logical Operator29/2
  [VDDM_ESC5RCErrDTC_cnt] -> Relay3/1
  Relay2/1 -> SR_Latch5/1
  [task_time_s] -> Test Detection Criteria4/2
  Logical Operator38/1 -> DTC_Couter4/1
  [VDDM_ESC5RCErrDet_flg] -> DTC_Info2/1
  [task_time_s] -> Test Detection Criteria3/2
  Logical Operator24/1 -> [VDDM_ESC5RCErrCFS_flg]  "VDDM_ESC5RCErrCFS_flg"
  Logical Operator4/1 -> [VDDM_ESC5NoComRst_flg], Switch3/3
  [VPMM_SysPwrSta_enum] -> Equal9/1
  Constant11/1 -> Equal14/2
  [No_CAN1_BUS_OFF] -> Logical Operator4/2
  Equal18/1 -> Logical Operator10/1
  Logical Operator12/1 -> Timer1/2
  Constant12/1 -> Switch1/1
  [task_time_s] -> Timer4/3
  Equal5/1 -> Logical Operator35/2
  Equal17/1 -> Logical Operator7/1
  Equal11/1 -> Logical Operator2/1
  DTC_Couter3/1 -> SR_Latch6/1
  Equal12/1 -> Logical Operator6/2
  Unit Delay3/1 -> Equal3/1
  SR_Latch9/1 -> Logical Operator40/1
  Equal14/1 -> Logical Operator7/2
  [DTC_clear_request] -> Switch1/2
  Constant52/1 -> Equal4/2
  [VDDM_ESC5NoComCFSRls_flg] -> Logical Operator14/1
  Logical Operator26/1 -> Logical Operator46/4
  Constant57/1 -> DTC_Couter3/3
  [VDDM_ESC5CSErrCFS_flg] -> DTC_Info3/3
  Constant1/1 -> Equal7/2
  Constant39/1 -> Logical Operator42/1
  [VDDM_ESC5CSErrDFSRls_flg] -> Logical Operator44/1
  Constant44/1 -> Test Detection Criteria4/4
  Logical Operator46/1 -> [VDDM_ESC5RCErrRst_flg], Switch1/3
  Logical Operator22/1 -> DTC_Couter3/1
  Logical Operator53/1 -> Logical Operator50/3
  Constant37/1 -> DTC_Couter4/3
  DTC_Couter4/2 -> Data Type Conversion4/1
  DTC_Couter3/2 -> Data Type Conversion1/1
  Constant9/1 -> DTC_Couter2/3
  DTC_Couter2/1 -> SR_Latch3/1
  Constant2/1 -> Equal9/2
  Logical Operator43/1 -> Timer4/1, Logical Operator37/1
  Unit Delay4/1 -> Equal22/1
  SR_Latch7/1 -> [VDDM_ESC5RCErrPass_flg]  "VDDM_ESC5RCErrPass_flg"
  Logical Operator19/1 -> Timer3/2
  Constant15/1 -> Equal17/2
  [VDDM_ESC5RCErr_flg] -> Logical Operator30/1
  Logical Operator41/1 -> Logical Operator32/4
  Timer4/1 -> Equal15/1
  Switch3/1 -> Test Detection Criteria2/1
  Logical Operator52/1 -> Logical Operator36/1
  [VDDM_ESC5CSErrDet_flg] -> Logical Operator38/1
  VDDM_ESC5NoCom_flg/1 -> [VDDM_ESC5NoCom_flg]
  [VDDM_ESC5NoComPass_flg] -> DTC_Info1/2
  [VDDM_ESC5NoCom_flg] -> Logical Operator53/1
  [No_CAN1_BUS_OFF] -> Logical Operator50/2
  [No_CAN1_BUS_OFF] -> Logical Operator32/2
  [VPMM_SysPwrSta_enum] -> Equal16/1
  SR_Latch11/1 -> Logical Operator42/2
  Test Detection Criteria3/1 -> [VDDM_ESC5RCErrDet_flg]  "VDDM_ESC5RCErrDet_flg"
  [VDDM_ESC5CSErrPass_flg] -> Logical Operator33/2
  [VDDM_ESC5RCErrCFSRls_flg] -> Logical Operator17/1
  Equal4/1 -> Logical Operator8/2
  DTC_Couter4/1 -> SR_Latch9/1
  Logical Operator37/1 -> Timer4/2
  SR_Latch5/1 -> Logical Operator48/2
  Constant54/1 -> Logical Operator21/2
  Test Detection Criteria2/1 -> [VDDM_ESC5NoComDet_flg]  "VDDM_ESC5NoComDet_flg"
  Constant34/1 -> Logical Operator23/2
  [VDDM_ESC5NoCom_flg] -> Logical Operator4/3
  Constant49/1 -> Equal3/2
  [VDDM_ESC5RCErrDFSRls_flg] -> Logical Operator29/1
  VDDM_ESC5RCErr_flg/1 -> [VDDM_ESC5RCErr_flg]
  VDDM_ESC5CSErr_flg/1 -> [VDDM_ESC5CSErr_flg]
  Logical Operator11/1 -> Logical Operator28/4
  [VDDM_ESC5NoComCFS_flg] -> Logical Operator11/1
  Logical Operator13/1 -> Logical Operator43/4
  [VDDM_ESC5NoComCFS_flg] -> Logical Operator13/1
  [VDDM_ESC5CSErrRst_flg] -> SR_Latch10/2
  [VDDM_ESC5NoComCFS_flg] -> VDDM_ESC5NoComCFS_flg/1
  [VDDM_ESC5RCErrCFS_flg] -> VDDM_ESC5RCErrCFS_flg/1
  [VDDM_ESC5CSErrCFS_flg] -> VDDM_ESC5CSErrCFS_flg/1
  Logical Operator15/1 -> Logical Operator20/3
  [DTC_clear_request] -> Logical Operator5/1, Logical Operator15/1
  [DTC_clear_request] -> Logical Operator14/2
  Logical Operator14/1 -> SR_Latch3/2
  [DTC_clear_request] -> Logical Operator51/3
  Logical Operator16/1 -> Logical Operator22/3
  [DTC_clear_request] -> Logical Operator47/1, Logical Operator16/1
  Logical Operator17/1 -> SR_Latch6/2
  [DTC_clear_request] -> Logical Operator17/2
  [DTC_clear_request] -> Logical Operator29/3
  Logical Operator18/1 -> Logical Operator38/3
  [DTC_clear_request] -> Logical Operator33/1, Logical Operator18/1
  Logical Operator34/1 -> SR_Latch9/2
  [DTC_clear_request] -> Logical Operator34/2
  [DTC_clear_request] -> Logical Operator44/3
